simulink model "test"  (R2022b)
settings: Solver=VariableStepAuto  StartTime=0.0  StopTime=inf  RelTol=1e-3
model workspace (MAT data in the model file):
  seed = 0.318765239859
  size = 100
settings Model: PauseTimes=0.001  PacingRate=0.001000  Creator=PSSENL  LastModifiedBy=rhdej

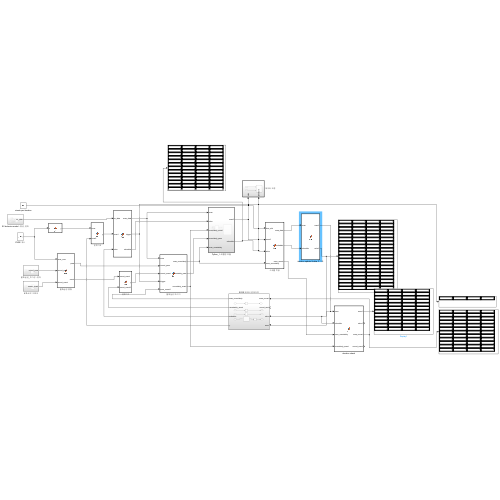
[thumbnail: Simulink's stored preview of the top-level diagram]
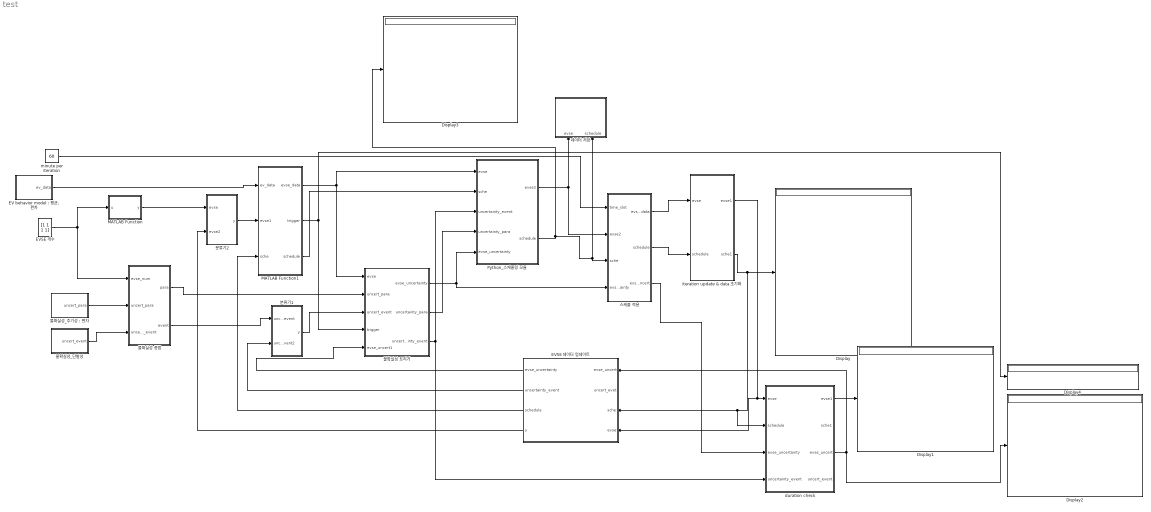
== system test ==
  Display{,1..4} (5 alike) : Display
  "EV behavior model : 평균, 편차" : Subsystem
  EVSE 개수 : Constant  Value=[1 1 1 1]
  EVSE 데이터 업데이트 : Subsystem
  MATLAB Function : MATLAB Function  TreatAsAtomicUnit=on
  MATLAB Function1 : MATLAB Function  TreatAsAtomicUnit=on
  Python_스케줄링 모듈 : Subsystem  TreatAsAtomicUnit=on
      settings: MinAlgLoopOccurrences=on
  duration check : MATLAB Function  TreatAsAtomicUnit=on
  iteration update & data 초기화 : MATLAB Function  TreatAsAtomicUnit=on
  minute per iteration : Constant  Value=60
  데이터 저장 : Subsystem  TreatAsAtomicUnit=on
      settings: MinAlgLoopOccurrences=on
  분류기1 : MATLAB Function  TreatAsAtomicUnit=on
  분류기2 : MATLAB Function  TreatAsAtomicUnit=on
  불확실성 종합 : MATLAB Function  TreatAsAtomicUnit=on
  불확실성 트리거 : MATLAB Function  TreatAsAtomicUnit=on
  불확실성_단발성 : Subsystem
  "불확실성_주기성 : 편차" : Subsystem
  스케줄 적용 : MATLAB Function  TreatAsAtomicUnit=on
  wires:
  EVSE 개수/1 -> 불확실성 종합/1(evse_num), MATLAB Function/1(u)
  분류기2/1(y) -> MATLAB Function1/2(evse1)
  MATLAB Function1/1(evse_data) -> 불확실성 트리거/1(evse), Python_스케줄링 모듈/1(evse)
  iteration update & data 초기화/2(sche1) -> duration check/2(schedule), EVSE 데이터 업데이트/3(sche), Display/1
  iteration update & data 초기화/1(evse1) -> EVSE 데이터 업데이트/4(evse), duration check/1(evse)
  MATLAB Function/1(y) -> 분류기2/1(evse)
  EVSE 데이터 업데이트/4(y) -> 분류기2/2(evse2)
  "EV behavior model : 평균, 편차"/1(ev_data) -> MATLAB Function1/1(ev_data)
  EVSE 데이터 업데이트/3(schedule) -> MATLAB Function1/3(sche)
  MATLAB Function1/3(schedule) -> Python_스케줄링 모듈/2(sche)
  Python_스케줄링 모듈/1(evse2) -> 데이터 저장/1(evse), 스케줄 적용/2(evse2)
  Python_스케줄링 모듈/2(schedule) -> 데이터 저장/2(schedule), 스케줄 적용/3(sche), Display3/1
  스케줄 적용/2(schedule) -> iteration update & data 초기화/2(schedule)
  스케줄 적용/1(evse_data) -> iteration update & data 초기화/1(evse)
  "불확실성_주기성 : 편차"/1(uncert_para) -> 불확실성 종합/2(uncert_para)
  불확실성_단발성/1(uncert_event) -> 불확실성 종합/3(uncert_event)
  불확실성 종합/1(para) -> 불확실성 트리거/2(uncert_para)
  불확실성 종합/2(event) -> 분류기1/1(uncert_event)
  MATLAB Function1/2(trigger) -> 불확실성 트리거/4(trigger), Display4/1
  불확실성 트리거/2(uncertainty_para) -> Python_스케줄링 모듈/4(uncertainty_para)
  minute per iteration/1 -> 스케줄 적용/1(time_slot)
  EVSE 데이터 업데이트/1(evse_uncertainty) -> 불확실성 트리거/5(evse_uncert1)
  EVSE 데이터 업데이트/2(uncertainty_event) -> 분류기1/2(uncert_event2)
  분류기1/1(y) -> 불확실성 트리거/3(uncert_event)
  스케줄 적용/3(evse_uncert) -> duration check/3(evse_uncertainty)
  duration check/1(evse1) -> Display1/1
  불확실성 트리거/3(uncertainty_event) -> Python_스케줄링 모듈/3(uncertainty_event), duration check/4(uncertainty_event)
  duration check/3(evse_uncert) -> Display2/1, EVSE 데이터 업데이트/1(evse_uncert)
  불확실성 트리거/1(evse_uncertainty) -> Python_스케줄링 모듈/5(evse_uncertainty), 스케줄 적용/4(evse_uncertainty)

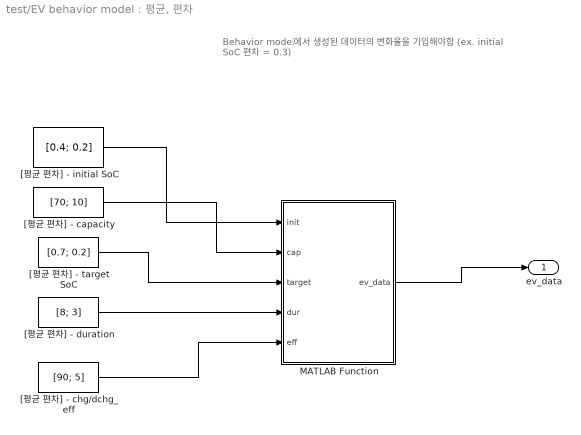
== system test/EV behavior model : 평균, 편차 ==
  note: Behavior model에서 생성된 데이터의 변화율을 기입해야함
      | (ex. initial SoC 편차 = 0.3)
  MATLAB Function : MATLAB Function  TreatAsAtomicUnit=on
  "[평균 편차] - capacity" : Constant  Value=[70; 10]
  "[평균 편차] - chg/dchg_eff" : Constant  Value=[90; 5]
  "[평균 편차] - duration" : Constant  Value=[8; 3]
  "[평균 편차] - initial SoC" : Constant  Value=[0.4; 0.2]
  "[평균 편차] - target SoC" : Constant  Value=[0.7; 0.2]
  ev_data : Outport
  wires:
  "[평균 편차] - initial SoC"/1 -> MATLAB Function/1(init)
  "[평균 편차] - capacity"/1 -> MATLAB Function/2(cap)
  "[평균 편차] - target SoC"/1 -> MATLAB Function/3(target)
  "[평균 편차] - duration"/1 -> MATLAB Function/4(dur)
  MATLAB Function/1(ev_data) -> ev_data/1
  "[평균 편차] - chg/dchg_eff"/1 -> MATLAB Function/5(eff)

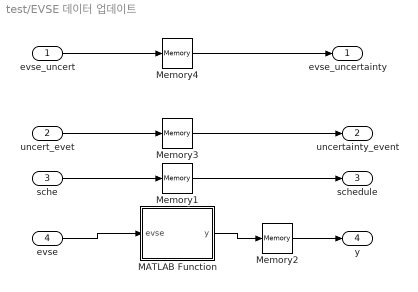
== system test/EVSE 데이터 업데이트 ==
  evse_uncert : Inport
  uncert_evet : Inport  Port=2
  sche : Inport  Port=3
  evse : Inport  Port=4
  MATLAB Function : MATLAB Function  TreatAsAtomicUnit=on
  Memory{1..4} (4 alike) : Memory
  evse_uncertainty : Outport
  uncertainty_event : Outport  Port=2
  schedule : Outport  Port=3
  y : Outport  Port=4
  wires:
  evse/1 -> MATLAB Function/1(evse)
  MATLAB Function/1(y) -> Memory2/1
  sche/1 -> Memory1/1
  Memory1/1 -> schedule/1
  Memory2/1 -> y/1
  evse_uncert/1 -> Memory4/1
  uncert_evet/1 -> Memory3/1
  Memory3/1 -> uncertainty_event/1
  Memory4/1 -> evse_uncertainty/1

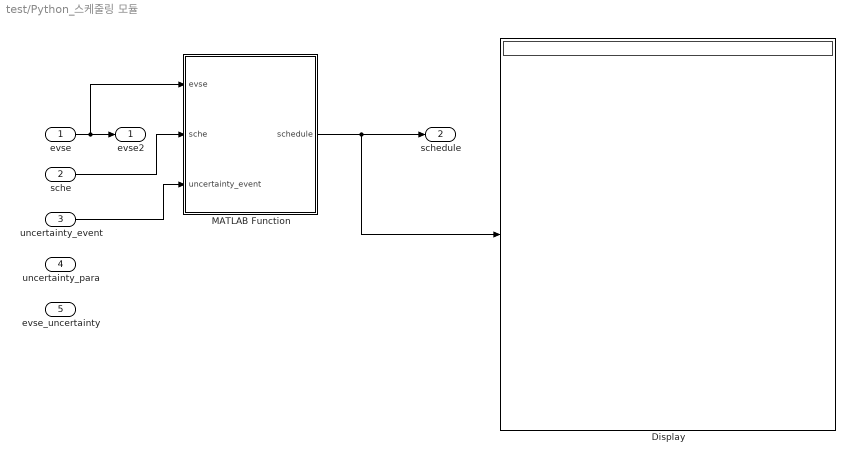
== system test/Python_스케줄링 모듈 ==
  evse : Inport
  sche : Inport  Port=2
  uncertainty_event : Inport  Port=3
  uncertainty_para : Inport  Port=4
  evse_uncertainty : Inport  Port=5
  Display : Display
  MATLAB Function : MATLAB Function  TreatAsAtomicUnit=on
  evse2 : Outport
  schedule : Outport  Port=2
  wires:
  MATLAB Function/1(schedule) -> Display/1, schedule/1
  sche/1 -> MATLAB Function/2(sche)
  evse/1 -> MATLAB Function/1(evse), evse2/1
  uncertainty_event/1 -> MATLAB Function/3(uncertainty_event)

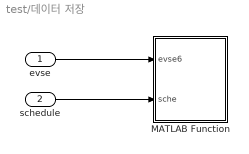
== system test/데이터 저장 ==
  evse : Inport
  schedule : Inport  Port=2
  MATLAB Function : MATLAB Function  TreatAsAtomicUnit=on
  wires:
  evse/1 -> MATLAB Function/1(evse6)
  schedule/1 -> MATLAB Function/2(sche)

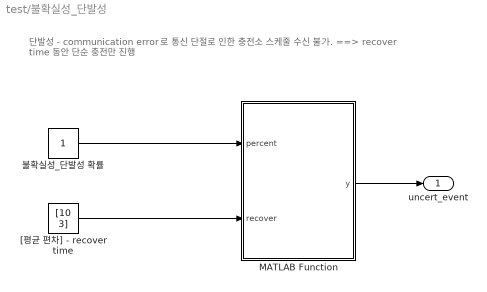
== system test/불확실성_단발성 ==
  note: 단발성 - communication error 로 통신 단절로 인한 충전소 스케줄 수신 불가.
      | ==> recover time 동안 단순 충전만 진행
  MATLAB Function : MATLAB Function  TreatAsAtomicUnit=on
  "[평균 편차] - recover time" : Constant  Value=[10 3]
  불확실성_단발성 확률 : Constant
  uncert_event : Outport
  wires:
  MATLAB Function/1(y) -> uncert_event/1
  "[평균 편차] - recover time"/1 -> MATLAB Function/2(recover)
  불확실성_단발성 확률/1 -> MATLAB Function/1(percent)

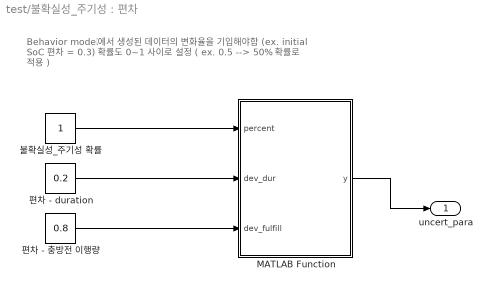
== system test/불확실성_주기성 : 편차 ==
  note: Behavior model에서 생성된 데이터의 변화율을 기입해야함
      | (ex. initial SoC 편차 = 0.3)
      | 확률도 0~1 사이로 설정 ( ex. 0.5 --> 50% 확률로 적용 )
  MATLAB Function : MATLAB Function  TreatAsAtomicUnit=on
  불확실성_주기성 확률 : Constant
  편차 - duration : Constant  Value=0.2
  편차 - 충방전 이행량 : Constant  Value=0.8
  uncert_para : Outport
  wires:
  편차 - duration/1 -> MATLAB Function/2(dev_dur)
  편차 - 충방전 이행량/1 -> MATLAB Function/3(dev_fulfill)
  MATLAB Function/1(y) -> uncert_para/1
  불확실성_주기성 확률/1 -> MATLAB Function/1(percent)

== matlab function test/불확실성_단발성/MATLAB Function ==
  data: y output; percent input; recover input
% 1: percent 2:recover mean 3: recover deviation
function y = fcn(percent, recover)

col = size(percent,1)+size(recover,1);
y = zeros(1,col);
y = [percent transpose(recover)];
end

== matlab function test/duration check ==
  data: evse input; evse1 output; schedule input; evse_uncertainty input; sche1 output; uncertainty_event input; evse_uncert output; uncert_event output
% 1 : state, 2:iteration 3: cap, 4: init, 5: target, 6: min, 7:max
% 8 : dur, 9: Pmin, 10: Pmax, 11 : chg_eff, 12: dchg_eff

% 1: init 2:cap 3:target 4:dur 5:eff

function [evse1,sche1,evse_uncert,uncert_event] = fcn(evse ,schedule, evse_uncertainty, uncertainty_event)
evse1 = zeros(12,size(evse,2));
state1 = zeros(12,size(evse,2)); % evse의 ev 모델
sche1 = zeros(25,size(schedule,2)); % evse별 스케줄
sche_data = zeros(25,size(schedule,2));
state2 = zeros(12,size(evse,2));

iter_evse = 0; % evse iteration
iter_sche = 0; % schedule iteration

if size(schedule,1) ~= 1
    sche_data = schedule;
end

if size(evse,1) ~= 1
    state1 = evse; % input
end

%% EVSE & schedule normal 버전
% evse iteration update
for i = 1:size(state1,2)
    if (state1(8,i) == 0)
        iter_evse = state1(2,i);
        state1(:,i) = 0;
        state1(2,i) = iter_evse;
        for j = 1:size(schedule,1)
            sche_data(j,i) = 0;
        end
    end
end

% schedule iteration update
for i = 1:size(state1,2)
    if (state1(1,i) == 1)
        iter_sche = sche_data(25,i);
        iter_sche = iter_sche + 1;
        sche_data(25,i) = iter_sche;
    end
end

%schedule matching with evse state
for i = 1:size(state1,2)
    if (size(schedule,1) == 25) && ((state1(1,i) == 0) || (state1(8,i) == 0))
        sche_data(25,i) = 0;
    end
end

%% 불확실성 duration check

if size(evse_uncertainty,1) ~= 1
    state2 = evse_uncertainty;
end

% para uncertainty update ( evse )
 % iteration
 for i = 1:size(evse,2)
     if (state2(8,i) == 0)
         iter_para = state2(2,i);
         state2(:,i) = 0;
         state2(2,i) = iter_para;
     end
 end

%%
evse1 = state1;
sche1 = sche_data;

evse_uncert = zeros(12,size(evse,2));
evse_uncert = state2;
uncert_event = uncertainty_event;

== matlab function test/불확실성 트리거 ==
  data: evse input; evse_uncertainty output; uncert_para input; uncert_event input; trigger input; uncertainty_para output; uncertainty_event output; evse_uncert1 input
% para - 1: percent 2: dur 3: fulfill
% event - 1: percent 2:recover mean 3: recover deviation

% 1 : state, 2:iteration 3: cap, 4: init, 5: target, 6: min, 7:max
% 8 : dur, 9: Pmin, 10: Pmax, 11 : chg_eff, 12: dchg_eff

function [evse_uncertainty,uncertainty_para, uncertainty_event] = fcn(evse, uncert_para, uncert_event, trigger, evse_uncert1)
coder.extrinsic("binornd", "randn", "rng")
rng shuffle

err_dur = zeros(1,size(evse,2)); % duration 오차율
err_eff = zeros(1,size(evse,2)); % efficiency 오차율
evse_uncert = zeros(12,size(evse,2)); % evse_data uncertainty version

uncert_para1 = zeros(3,size(evse,2));
uncert_event1 = zeros(3,size(evse,2));

state_para = zeros(1,size(evse,2)); % 주기성 상태
state_event = zeros(1,size(evse,2)); % event state

%% 트리거 변수에 따른 스케줄링 불확실성 적용버전 생성
for i = 1:size(evse,2)
    % parameter uncertainty generation
    % EV model generation check
    if trigger(1,i) == 1
        % uncertainty generation
        state_para(1,i) = binornd(1,uncert_para(1,i));
        % uncertainty generation check
        if state_para(1,i) == 1
            %duration
            dur = 0;
            dur = randn * uncert_para(2,i);
            
            % 무조건 음수로
            if dur > 0
                dur = -dur;
            end
            err_dur(1,i) = dur;
                       
            % efficiency
            eff = 0;
            eff = randn * uncert_para(3,i);

            % 무조건 음수로
            if eff > 0
                eff = -eff;
            end
            err_eff(1,i) = eff;
            
            % EVSE 적용
            evse_uncert = evse;
            evse_uncert(8,i) = floor(evse_uncert(8,i) * (1 + err_dur(1,i))); % duration
            evse_uncert(11,i) = floor(evse_uncert(11,i) * (1 + err_eff(1,i))); % chg_eff
            evse_uncert(12,i) = evse_uncert(11,i);
        end

    elseif (trigger(1,i) == 0) && (size(evse_uncert1,1) ~= 1)
        for j = 1:12
            evse_uncert(j,i) = evse_uncert1(j,i);
        end
    end
        uncert_para1(1,i) = state_para(1,i);
        uncert_para1(2,i) = err_dur(1,i);
        uncert_para1(3,i) = err_eff(1,i);
        trigger(1,i) = 0;
end

    % event ucnertainty generation
    event_state = 0;
    event_state = binornd(1,uncert_event(1,i));
    uncert_event1(2,i) = event_state;
    % event state check
    if state_event(1,i) == 1
        t = 0;
        t = uncert_event(3,i) * randn;
        data_recover = 0;
        data_recover = uncert_event(2,i) + t;
        uncert_event1(3,i) = data_recover;
    end
    uncert_event1(1,i) = uncert_event1(1,i) + 1;

% event - 1: iteration 2: state 3: recover

evse_uncertainty = zeros(12,size(evse,2));

uncertainty_para = uncert_para1;
uncertainty_event = uncert_event1;
evse_uncertainty = evse_uncert;

== matlab function test/분류기1 ==
  data: y output; uncert_event input; uncert_event2 input
% 1 : state, 2:iteration 3: cap, 4: init, 5: target, 6: min, 7:max
% 8 : dur, 9: Pmin, 10: Pmax, 11 : chg_eff, 12: dchg_eff

function y = fcn(uncert_event, uncert_event2)
coder.extrinsic("delete")

event_data = zeros(size(uncert_event));
event_data = uncert_event;


% evse 데이터 분류
if size(uncert_event2) == size(uncert_event)
    event_data = uncert_event2;
end

% 이전 시뮬레이션 결과 삭제
    
for i = 1:size(uncert_event,2)
    if event_data(1,i) == 0
        txt1 = sprintf('result/state/uncert_event_%d.csv',int8(i));
%         txt2 = sprintf('result/normal/schedule_%d.csv',int8(i));
        delete(txt1);
%         delete(txt2);
    end
end

y = zeros(size(uncert_event));
y = event_data;

== matlab function test/데이터 저장/MATLAB Function ==
  data: evse6 input; sche input
% 1 : state, 2:iteration 3: cap, 4: init, 5: target, 6: min, 7:max
% 8 : dur, 9: Pmin, 10: Pmax, 11 : chg_eff, 12: dchg_eff

function fcn(evse6, sche)
coder.extrinsic("writematrix")
coder.extrinsic("readmatrix")
coder.extrinsic("int8")
coder.extrinsic("exist")

evse_num = size(evse6,2);
iter_sche = 0;
a = 0;
b = 0;
row_num = 0;
row_num_sche = 0;

% evse 저장
for i = 1:evse_num
    txt1 = sprintf('result/evse_%d.csv',int8(i));
    a = exist(txt1);
    if a == 0
        ev_data = zeros(1,size(evse6,1));
        writematrix(ev_data,txt1);
        data_evse1 = readmatrix(txt1);
        data_evse2 = zeros(row_num + 1,12);
        data_evse2 = vertcat(data_evse1, transpose(evse6(:,i)));
        writematrix(data_evse2,txt1);
    else
        data_evse1 = readmatrix(txt1);
        row_num = size(data_evse1,1);
        data_evse2 = zeros(row_num + 1,12);
        data_evse2 = vertcat(data_evse1, transpose(evse6(:,i)));
        writematrix(data_evse2,txt1);
    end
end
    
% schedule 저장
for i = 1:evse_num
    txt2 = sprintf('result/schedule_%d.csv',int8(i));
    b = exist(txt2);
    iter_sche = sche(25,i);
    if b == 0
        for j = 1 : size(sche,1)
            data_sche = zeros(1,size(sche,1));
            data_sche3 = zeros(2,size(sche,1));
            writematrix(data_sche3,txt2);
            data_sche(1,1:iter_sche) = sche(1:iter_sche,i);
            data_sche2 = zeros(row_num_sche+1,size(sche,1));
            data_sche3 = vertcat(data_sche3,data_sche);
            writematrix(data_sche,txt2);
        end
    else
        data_sche5 = readmatrix(txt2);
        row_num_sche = size(data_sche5,1);
        data_sche3 = zeros(row_num_sche + 1,size(sche,1));
        data_sche4 = zeros(1,size(sche,1));
        for j = 1:size(sche,1)
            data_sche4(1,1:iter_sche) = sche(1:iter_sche,i);
            if j == 25
                data_sche4(1,j) = sche(j,i);
            end
        end
        data_sche3 = vertcat(data_sche5,data_sche4);
        writematrix(data_sche3,txt2);
    end
end

== matlab function test/분류기2 ==
  data: y output; evse input; evse2 input
% 1 : state, 2:iteration 3: cap, 4: init, 5: target, 6: min, 7:max
% 8 : dur, 9: Pmin, 10: Pmax, 11 : chg_eff, 12: dchg_eff

function y = fcn(evse, evse2)
coder.extrinsic("delete")

evse_data = zeros(size(evse));
evse_data = evse;

% evse 데이터 분류
if size(evse2,1) == 12
    evse_data = evse2;
end
% 이전 시뮬레이션 결과 삭제
    
for i = 1:size(evse,2)
    if evse_data(2,i) == 0
        txt1 = sprintf('result/evse_%d.csv',int8(i));
        txt2 = sprintf('result/schedule_%d.csv',int8(i));
        delete(txt1);
        delete(txt2);
    end
end

y = zeros(size(evse));
y = evse_data;

== matlab function test/iteration update & data 초기화 ==
  data: evse input; evse1 output; schedule input; sche1 output
% 1 : state, 2:iteration 3: cap, 4: init, 5: target, 6: min, 7:max
% 8 : dur, 9: Pmin, 10: Pmax, 11 : chg_eff, 12: dchg_eff

% 1: init 2:cap 3:target 4:dur 5:eff

function [evse1,sche1] = fcn(evse ,schedule)
state1 = zeros(size(evse)); % evse의 ev 모델
evse1 = zeros(12,size(evse,2)); % evse output
sche1 = zeros(25,size(schedule,2)); % evse별 스케줄
sche_data = zeros(25,size(schedule,2));
sche_data = schedule;

iter_evse = 0; % evse iteration
iter_sche = 0; % schedule iteration

state1 = evse; % input

% evse iteration update
for i = 1:size(state1,2)
    if (state1(8,i) == 0)
        iter_evse = state1(2,i);
        state1(:,i) = 0;
        state1(2,i) = iter_evse;
        for j = 1:25
            sche_data(j,i) = 0;
        end
    end
end

% schedule iteration update
for i = 1:size(state1,2)
    if (state1(1,i) == 1)
        iter_sche = sche_data(25,i);
        iter_sche = iter_sche + 1;
        sche_data(25,i) = iter_sche;
    end
end


%schedule matching with evse state
for i = 1:size(state1,2)
    if (25 == 25) && ((state1(1,i) == 0) || (state1(8,i) == 0))
        sche_data(25,i) = 0;
    end
end


evse1 = state1;
sche1 = sche_data;

== matlab function test/MATLAB Function ==
  data: u input; y output [1..100]
function y = fcn(u)
% 1 : state, 2:iteration 3: cap, 4: init, 5: target, 6: min, 7:max
% 8 : dur, 9: Pmin, 10: Pmax, 11 : chg_eff, 12: dchg_eff
coder.extrinsic("delete")

num_cols = size(u, 1);
y = zeros(12, num_cols);

== matlab function test/스케줄 적용 ==
  data: time_slot input; evse2 input; evse_data output; sche input; schedule output; evse_uncertainty input; evse_uncert output
% 1 : state, 2:iteration 3: cap, 4: init, 5: target, 6: min, 7:max
% 8 : dur, 9: Pmin, 10: Pmax, 11 : chg_eff, 12: dchg_eff

% 1: init 2:cap 3:target 4:dur 5:eff
function [evse_data,schedule, evse_uncert] = fcn(time_slot, evse2, sche, evse_uncertainty)
coder.extrinsic('round')
coder.extrinsic('rng')
coder.extrinsic('randn')

rng('shuffle');

state = zeros(12,size(evse2,2)); % evse data
state = evse2;

state2 = zeros(12,size(evse2,2)); % evse uncertainty data
state2 = evse_uncertainty;

iter_sche = 0; % schedule iteration
iter_sche2 = 0;

%% 데이터 업데이트 및 check
%duration
for i = 1:size(state,2)
    state(2,i) = state(2,i) + 1; % iteration
    if (state(1,i) == 1) && (state(3,i) ~= 0)
        % schedule update
        if size(sche,1) == 25
            iter_sche = sche(25,i);
            if (state(8,i) ~= 0) && (iter_sche ~= 0)
                % schedule - initial SoC
                %chg
                if (sche(iter_sche,i) >= 0)
                    state(4,i) = round((state(4,i) * state(3,i) + sche(iter_sche,i)*(time_slot/60))*(state(11,i)/100)/state(3,i),2);
                else
                    %dchg
                    state(4,i) = round((state(4,i) * state(3,i) + sche(iter_sche,i)*(time_slot/60))*(state(12,i)/100)/state(3,i),2);
                end
%                 sche(25,i) = sche(25,i) + 1; % schedule iteration update
            end
        end
        % duration
        state(8,i) = state(8,i) - 1;
    end

    % 불확실성 버전도 schedule 적용
    state2(2,i) = state(2,i);
    
    if (state2(1,i) == 1) && (state2(3,i) ~= 0)
        if size(sche,1) == 25
            iter_sche2 = 0;
            iter_sche2 = sche(25,i);
            if (state2(8,i) ~= 0) && (iter_sche2 ~= 0)
                if (sche(iter_sche2,i) >= 0)
                    state2(4,i) = round((state2(4,i) * state2(3,i) + sche(iter_sche2,i)*(time_slot/60))*(state2(11,i)/100)/state2(3,i),2);
                else
                    state2(4,i) = round((state2(4,i) * state2(3,i) + sche(iter_sche2,i)*(time_slot/60))*(state2(12,i)/100)/state2(3,i),2);
                end
            end
        end
    end
end

schedule = zeros(25,size(sche,2));
evse_data = zeros(12,size(evse2,2));
evse_uncert = zeros(12,size(evse2,2));

schedule = sche;
evse_data = state;
evse_uncert = state2;

== matlab function test/EVSE 데이터 업데이트/MATLAB Function ==
  settings: updateMethod=DISCRETE
  data: evse input; y output
function y= fcn(evse)
coder.extrinsic("round","binornd","rng")

rng shuffle

% 운용 가능 플러그 개수 확인하기
idx = find(evse(1,:)==0);
empty_num = size(find(evse(1,:) == 0),2);

% 운용 가능 플러그 개수만큼 분포 발생하기
if sum(empty_num) ~= 0
   for i = 1:empty_num
       evse(1,idx(i)) = binornd(1,0.5);
   end
end

y = evse;

== matlab function test/EV behavior model : 평균, 편차/MATLAB Function ==
  data: init input; ev_data output; cap input; target input; dur input; eff input
% 1: init 2:cap 3:target 4:dur 5:eff
function ev_data = fcn(init, cap, target, dur, eff)
ev_data = [init cap target dur eff];

end

== matlab function test/MATLAB Function1 ==
  data: evse_data output; trigger output; ev_data input; evse1 input; sche input; schedule output
% 1 : state, 2:iteration 3: cap, 4: init, 5: target, 6: min, 7:max
% 8 : dur, 9: Pmin, 10: Pmax, 11 : chg_eff, 12: dchg_eff

% 1: init 2:cap 3:target 4:dur 5:eff

function [evse_data, trigger, schedule] = fcn(ev_data, evse1, sche)
coder.extrinsic('round')
coder.extrinsic('rng')
coder.extrinsic('randn')

rng('shuffle');

state = zeros(12,size(evse1,2)); % evse data
state = evse1;
trigger1 = zeros(1,size(evse1,2));
trigger = zeros(1,size(evse1,2));

%% evse 상태에 따라 정규분포로 데이터 생성
for i = 1:size(state,2)
    if (state(1,i) == 1) && (state(3,i) == 0)
        cap = 0;
        cap = ev_data(2,2)*randn;
        state(3,i) = round(ev_data(1,2) + cap,1);%capacity

        init = 0;
        init = ev_data(2,1)*randn;
        state(4,i) = round(ev_data(1,1) + init,1); % initial SoC

        target = 0;
        target = ev_data(2,3)*randn;
        state(5,i) = round(ev_data(1,3) + target,2); % target SoC
        state(6,i) = 0.05; % min
        state(7,i) = 0.95; % max
        
        dur = 0;
        dur = ev_data(2,4)*randn;
        state(8,i) = round(ev_data(1,4)+dur); % duration
        state(9,i) = -5; %Pmin
        state(10,i) = 11; %Pmax

        eff = 0;
        eff = ev_data(2,5)*randn;
        state(11,i) = round(ev_data(1,5)+eff); %chg_eff
        state(12,i) = state(11,i); %dchg_eff

        % SoC boundary
        if (state(4,i) < 0) || (state(4,i) > 0.6)
            state(4,i) = 0.2;
        end

        if (state(5,i) >= 1)
            state(5,i) = 0.8;
        end

        %duration minus
        if state(8,i) <= 0
            state(8,i) = 2;
        end

        if state(11,i) >= 100
            state(11,i) = 99;
        end

        state(12,i) = state(11,i); %dchg_eff
        trigger1(1,i) = 1;
    end
end
schedule = zeros(25,size(sche,2));
evse_data = zeros(size(evse1));

trigger = trigger1;
schedule = sche;
evse_data = state;

== matlab function test/불확실성_주기성 : 편차/MATLAB Function ==
  data: percent input; y output; dev_dur input; dev_fulfill input
% 1: percent 2:dur 3:fulfill
function y = fcn(percent, dev_dur, dev_fulfill)

col = size(dev_dur,1)+size(dev_fulfill,1)+size(percent,1);
y = zeros(1,col);
y = [percent dev_dur dev_fulfill];
end

== matlab function test/불확실성 종합 ==
  settings: updateMethod=DISCRETE
  data: para output [1..100]; evse_num input; uncert_para input; uncert_event input; event output
% para - 1: percent 2: dur 3: fulfill
% event - 1: percent 2:recover mean 3: recover deviation

function [para,event] = fcn(evse_num, uncert_para, uncert_event)

col = size(evse_num,1);
row_para = size(uncert_para,2);
row_event = size(uncert_event,2);

para1 = zeros(row_para,col);
event1 = zeros(row_event,col);

for i = 1:col
    para1(:,i) = uncert_para(1,:);
    event1(:,i) = uncert_event(1,:);
end

para = para1;
event = event1;

== matlab function test/Python_스케줄링 모듈/MATLAB Function ==
  data: evse input; schedule output; sche input; uncertainty_event input
% event - 1: iteration 2: state 3: recover

function schedule = fcn(evse, sche, uncertainty_event)
coder.extrinsic("writematrix")
coder.extrinsic("readmatrix")

sche_sample = readmatrix("input/sample schedule.csv");
evse_num = size(evse,2);
sche_data1 = zeros(25,evse_num);
schedule = zeros(25,evse_num);

% EVSE 상태에 따른 스케줄 생성
for i = 1:evse_num
    if (evse(1,i) == 1) && (evse(3,i) ~= 0) % state check
        for j = 1 : 24
            sche_data1(j,i) = sche_sample(j,i); % schedule 생성
            sche_data1(25,i) = 1;

            % event - communication error --> dumb charging
            if (uncertainty_event(1,i) ~= 0) && (uncertainty_event(2,i) == 1) && (uncertainty_event(3,i) ~= 0)
                sche_data1(j,i) = 8;
            end
        end
    end
end
% schedule iteration check
if size(sche,1) == 25
    for i = 1:evse_num
        iter_sche = sche(25,i);
        if iter_sche == 0
            sche_data1(25,i) = 1;
        else
            sche_data1(25,i) = sche(25,i);
        end
        if evse(1,i) == 0
            sche_data1(25,i) = 0;
        end
    end
end

schedule = sche_data1;
